simulink library "Lib_PFSys_GeneralDCDCConv_TMATS"  (R2020b)
settings: Solver=ode45  StartTime=0.0  StopTime=10.0  RelTol=1e-3  EnableMultiTasking=on
libraries: Lib_PF_BusLoadDC_TMATS x1, Lib_PF_ActiveConvEffDC2DC_TMATS x1
Description:
  | Thomas Modules
settings Model: Creator=jwchapm2  LastModifiedBy=mebell
settings DataIOCC: LimitDataPoints=on  SaveFormat=Array  ReturnWorkspaceOutputs=off
settings OptimizationCC: ExpressionDepthLimit=2147483647  LifeSpan=inf
settings DebuggingCC: UnderspecifiedInitializationDetection=Classic  MergeDetectMultiDrivingBlocksExec=none  SolverPrmCheckMsg=warning  StateNameClashWarn=warning  SFUnexpectedBacktrackingDiag=warning  SFNoUnconditionalDefaultTransitionDiag=warning  SFExecutionAtInitializationDiag=none  ArithmeticOperatorsInVariantConditions=warning
settings HardwareCC: ProdBitPerPointer=32  ProdBitPerSizeT=32  ProdBitPerPtrDiffT=32  ProdLargestAtomicFloat=None  ProdIntDivRoundTo=Undefined  ProdEndianess=Unspecified  ProdWordSize=32  ProdHWDeviceType=32-bit Generic
settings ModelReferenceCC: PropagateSignalLabelsOutOfModel=off
settings SFSimCC: SimUseLocalCustomCode=off  CustomCodeUndefinedFunction=UseInterfaceOnly
settings RTWCC: RTWUseLocalCustomCode=off
settings CodeAppCC: StateflowObjectComments=on
settings GRTTargetCC: TargetLangStandard=C89/C90 (ANSI)
settings ConfigComp: CovMetricSettings=dw  CovSaveCumulativeToWorkspaceVar=on  CovSaveSingleToWorkspaceVar=on  CovExternalEMLEnable=off

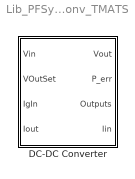
== system Lib_PFSys_GeneralDCDCConv_TMATS ==
  DC-DC Converter : Subsystem  mask(DC-DC Converter){X_C_VoltageVec_M=[0.0 0.1 1.0], Y_C_CurrentVec_M=[0.0 0.1 1.0], T_C_EffArray_M=[0.5 0.5 0.5; 0.5 1.0 1.0; 0.5 1.0 1.0], Pdis_M=1}
      mask prompts: X_C_VoltageVec_M "X_C_VoltageVec_M - Efficiency Table Voltage Vector (X-axis)(nx1), V"; Y_C_CurrentVec_M "Y_C_CurrentVec_M - Efficiency Table Current Vector (Y-axis)(mx1), A"; T_C_EffArray_M "T_C_EffArray_M - Efficiency Table Values (Eff = f(i, V)(nxm), Frac"; Pdis_M "Pdis_M - Constant Power Leaked/Dissipated, W"
      mask help:
      | This block represents a generic DC-DC converter controlled to produce a
      | constant output voltage (either a buck, boost, buck-boost, Cuk, etc.).
      | The converter's efficiency is defined via a lookup table that is a function
      | of input voltage and current. The input current is solved for, such that
      | the power in equals the power out.

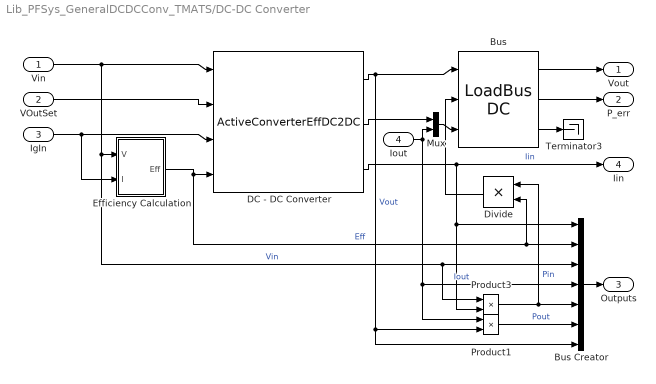
== system Lib_PFSys_GeneralDCDCConv_TMATS/DC-DC Converter ==
  Vin : Inport
  VOutSet : Inport  Port=2
  IgIn : Inport  Port=3
  Iout : Inport  Port=4
  Bus : Lib_PF_BusLoadDC_TMATS/LoadBus DC  P_M=-Pdis_M  BlkNm_M=double(gcb)
  Bus Creator : BusCreator  Inputs=7
  DC - DC Converter : Lib_PF_ActiveConvEffDC2DC_TMATS/ActiveConverterEffDC2DC  BlkNm_M=double(gcb)
  Divide : Product  Inputs=**
  Efficiency Calculation : Subsystem
  Mux : Mux  Inputs=2
  Product1 : Product
  Product3 : Product
  Terminator3 : Terminator
  Vout : Outport
  P_err : Outport  Port=2
  Outputs : Outport  Port=3
  Iin : Outport  Port=4
  wires:
  Bus/1 -> Vout/1
  Product1/1 -> Bus Creator/6  "Pout"
  Product3/1 -> Divide/1, Bus Creator/5  "Pin"
  Bus Creator/1 -> Outputs/1
  Efficiency Calculation/1(Eff) -> DC - DC Converter/4, Divide/2, Bus Creator/2  "Eff"
  Iout/1 -> Bus Creator/4, Product1/1, Mux/2  "Iout"
  Vin/1 -> DC - DC Converter/1, Bus Creator/3, Product3/1, Efficiency Calculation/1(V)  "Vin"
  IgIn/1 -> DC - DC Converter/3, Efficiency Calculation/2(I)
  VOutSet/1 -> DC - DC Converter/2
  DC - DC Converter/2 -> Mux/1
  DC - DC Converter/3 -> Product3/2, Bus Creator/1, Iin/1  "Iin"
  DC - DC Converter/1 -> Bus/1, Bus Creator/7, Product1/2  "Vout"
  Mux/1 -> Bus/3
  Bus/3 -> Terminator3/1
  Bus/2 -> P_err/1
  Divide/1 -> Bus/2

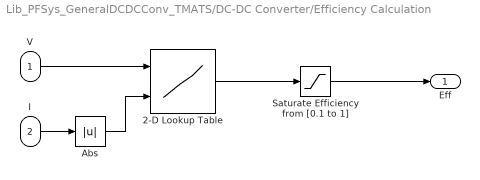
== system Lib_PFSys_GeneralDCDCConv_TMATS/DC-DC Converter/Efficiency Calculation ==
  V : Inport
  I : Inport  Port=2
  2-D Lookup Table : Lookup_n-D  BreakpointsForDimension1=X_C_VoltageVec_M  BreakpointsForDimension2=Y_C_CurrentVec_M  Table=T_C_EffArray_M  ExtrapMethod=Clip  InternalRulePriority=Speed  RndMeth=Simplest  InputSameDT=on
      settings: InputPortMap=u0,u1
  Abs : Abs
  Saturate Efficiency from [0.1 to 1] : Saturate  UpperLimit=1  LowerLimit=0.1
  Eff : Outport
  wires:
  Saturate Efficiency from [0.1 to 1]/1 -> Eff/1
  V/1 -> 2-D Lookup Table/1
  Abs/1 -> 2-D Lookup Table/2
  I/1 -> Abs/1
  2-D Lookup Table/1 -> Saturate Efficiency from [0.1 to 1]/1
